simulink model "sist_elect_simulink"  (R2024b)
settings: Solver=VariableStepAuto  StartTime=0.0  StopTime=10  RelTol=1e-3
InitFcn:
  |     Ra = 2;     %Ohms
  |     Kt = 0.01;  %Vs/Rad
  |     b = 0.0012; %Nms/Rad
  |     La = 0.023; %H
  |     Ke = 0.01;  %Vs/Rad
  |     J = 0.001;  %Kgm^2
settings Model: Creator=PC WHALE

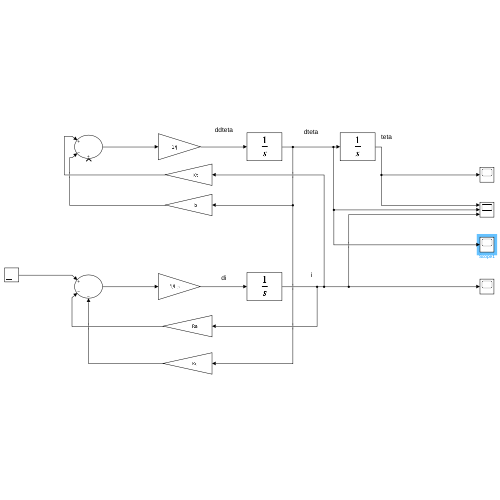
[thumbnail: Simulink's stored preview of the top-level diagram]
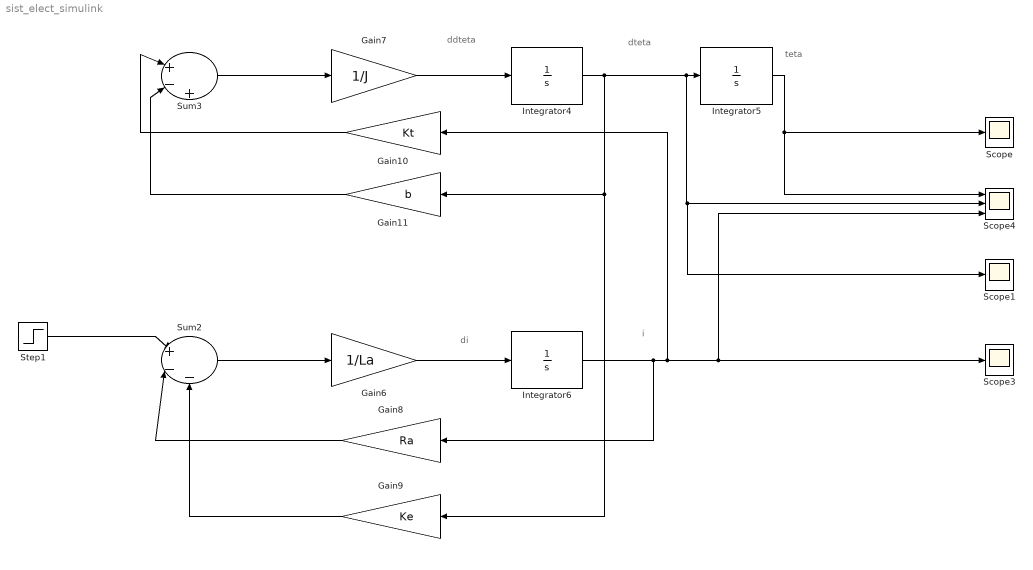
== system sist_elect_simulink ==
  note: ddteta
  note: dteta
  note: teta
  note: di
  note: i
  Gain10 : Gain  Gain=Kt
  Gain11 : Gain  Gain=b
  Gain6 : Gain  Gain=1/La
  Gain7 : Gain  Gain=1/J
  Gain8 : Gain  Gain=Ra
  Gain9 : Gain  Gain=Ke
  Integrator4 : Integrator
  Integrator5 : Integrator
  Integrator6 : Integrator
  Scope : Scope
  Scope1 : Scope
  Scope3 : Scope
  Scope4 : Scope  NumInputPorts=3
  Step1 : Step  Time=0  After=5  SampleTime=0
  Sum2 : Sum  Inputs=|+--
  Sum3 : Sum  Inputs=|+-+
  wires:
  Sum3/1 -> Gain7/1
  Sum2/1 -> Gain6/1
  Gain6/1 -> Integrator6/1
  Gain7/1 -> Integrator4/1
  Integrator4/1 -> Gain9/1, Gain11/1, Scope1/1, Scope4/2, Integrator5/1
  Integrator6/1 -> Gain10/1, Scope4/3, Scope3/1, Gain8/1
  Gain9/1 -> Sum2/3
  Gain8/1 -> Sum2/2
  Gain10/1 -> Sum3/1
  Gain11/1 -> Sum3/2
  Integrator5/1 -> Scope4/1, Scope/1
  Step1/1 -> Sum2/1
